simulink model "DZ_DSMC4"  (R2021b)
settings: Solver=FixedStepAuto  StartTime=0.0  StopTime=30  FixedStep=Ts  MaxStep=0.015  RelTol=1e-3  EnableMultiTasking=on
PreLoadFcn:
  | if ~exist('sim_HIL')
  |     sim_HIL=false;
  | end
  | if ~exist('usefilter')
  |     usefilter=false;
  | end
InitFcn:
  | load motorModel.mat
  | load expsetup
undefined symbols (not defined in the file): Cs, dels, etas, gamms, mModel, N, qTs, Ts, vphis, xiTs
settings Model: DataDictionary=MotorInfo.sldd  CodeVerificationMode=processor-in-the-loop (pil)  ExtModeTrigDuration=2  Creator=khoi  LastModifiedBy=khoi
settings SolverCC: AlgebraicLoopSolver=TrustRegion
settings DataIOCC: ExternalInput=i1, i2  SaveOutput=off  SaveTime=off
settings OptimizationCC: UseDivisionForNetSlopeComputation=on  GainParamInheritBuiltInType=on  UseFloatMulNetSlope=on  DefaultUnderspecifiedDataType=single  StrengthReduction=on  BitwiseOrLogicalOp=Bitwise operator  PassReuseOutputArgsAs=Individual arguments  ZeroExternalMemoryAtStartup=off  ZeroInternalMemoryAtStartup=off  EfficientFloat2IntCast=on  LifeSpan=1  MaxStackSize=64  OptimizeBlockOrder=speed  OptimizationPriority=Speed  OptimizationCustomize=off  MultiThreadedLoops=on  EfficientTunableParamExpr=on
settings DebuggingCC: SignalInfNanChecking=error  AlgebraicLoopMsg=none  ParameterTunabilityLossMsg=error  UniqueDataStoreMsg=error  AssertControl=DisableAll  StrictBusMsg=ErrorOnBusTreatedAsVector  SFUndirectedBroadcastEventsDiag=error  SFMachineParentedDataDiag=warning
settings HardwareCC: ProdBitPerInt=16  ProdBitPerPointer=16  ProdBitPerSizeT=16  ProdBitPerPtrDiffT=16  ProdLargestAtomicFloat=None  ProdWordSize=8  ProdHWDeviceType=Atmel->AVR
settings ModelReferenceCC: PropagateVarSize=During execution
settings SFSimCC: CompileTimeRecursionLimit=0  EnableRuntimeRecursion=off  MATLABDynamicMemAlloc=off
settings RTWCC: Description=Embedded Coder  SystemTargetFile=ert.tlc  HardwareBoard=Arduino Mega 2560  TemplateMakefile=ert_default_tmf  Toolchain=Arduino AVR  BuildConfiguration=Faster Runs
settings CodeAppCC: ForceParamTrailComments=on  IgnoreCustomStorageClasses=off  IgnoreTestpoints=on  OperatorAnnotations=on  SimulinkDataObjDesc=on  SFDataObjDesc=on  MATLABFcnDesc=on  InsertBlockDesc=on
settings ERTTargetCC: TargetLangStandard=C99 (ISO)  CodeReplacementLibrary=GNU C99 extensions  UtilityFuncGeneration=Shared location  SupportNonFinite=off  SupportComplex=off  ParenthesesLevel=Maximum  CastingMode=Standards  GenerateSharedConstants=off  ExtModeTransport=3  ExtModeStaticAlloc=on  ExtModeStaticAllocSize=2048  ExtModeMexFile=ext_xcp  ExtModeIntrfLevel=Level2 - Open  EnableSignedLeftShifts=off  EnableSignedRightShifts=off
settings ConfigComp: CovScope=ReferencedModels

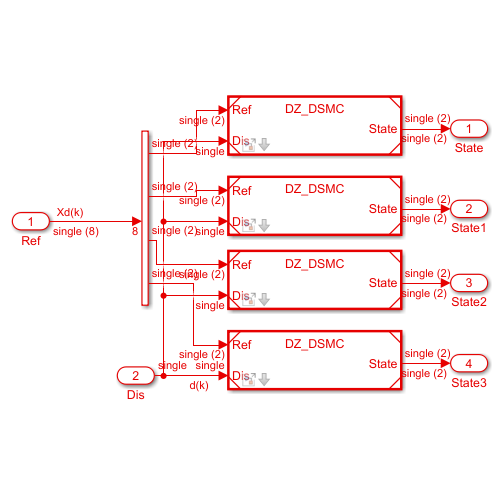
[thumbnail: Simulink's stored preview of the top-level diagram]
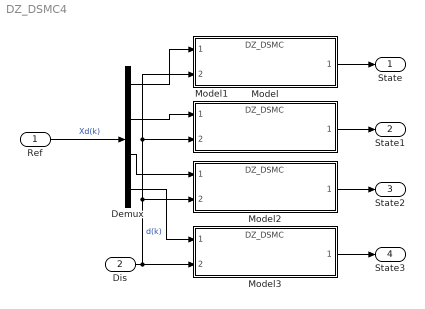
== system DZ_DSMC4 ==
  Ref : Inport  OutDataTypeStr=single  PortDimensions=8
  Dis : Inport  Port=2  OutDataTypeStr=single  PortDimensions=1
  Demux : Demux
  Model : ModelReference  ModelNameDialog=DZ_DSMC.slx  SimulationMode=Normal  ModelReferenceVersion=4.50  mask{Phi=mModel{1,3}.A, Gam=mModel{1,3}.B, C=Cs(1,:), qT=qTs(1), xiT=xiTs(1), del=dels(1), vphi=vphis(1), gamm=gamms(1), eta=etas(1), Ts=Ts, N=N}
      mask prompts: Phi "state A"; Gam "state B"; C "Sliding vector"; del "delta"; gamm "gamma"
  Model1 : ModelReference  ModelNameDialog=DZ_DSMC.slx  SimulationMode=Normal  ModelReferenceVersion=4.50  mask{Phi=mModel{2,3}.A, Gam=mModel{2,3}.B, C=Cs(2,:), qT=qTs(2), xiT=xiTs(2), del=dels(2), vphi=vphis(2), gamm=gamms(2), eta=etas(2), Ts=Ts, N=N}
      mask prompts: Phi "state A"; Gam "state B"; C "Sliding vector"; del "delta"; gamm "gamma"
  Model2 : ModelReference  ModelNameDialog=DZ_DSMC.slx  SimulationMode=Normal  ModelReferenceVersion=4.50  mask{Phi=mModel{3,3}.A, Gam=mModel{3,3}.B, C=Cs(3,:), qT=qTs(3), xiT=xiTs(3), del=dels(3), vphi=vphis(3), gamm=gamms(3), eta=etas(3), Ts=Ts, N=N}
      mask prompts: Phi "state A"; Gam "state B"; C "Sliding vector"; del "delta"; gamm "gamma"
  Model3 : ModelReference  ModelNameDialog=DZ_DSMC.slx  SimulationMode=Normal  ModelReferenceVersion=4.50  mask{Phi=mModel{4,3}.A, Gam=mModel{4,3}.B, C=Cs(4,:), qT=qTs(4), xiT=xiTs(4), del=dels(4), vphi=vphis(4), gamm=gamms(4), eta=etas(4), Ts=Ts, N=N}
      mask prompts: Phi "state A"; Gam "state B"; C "Sliding vector"; del "delta"; gamm "gamma"
  State : Outport  OutDataTypeStr=single  PortDimensions=2
  State1 : Outport  Port=2  OutDataTypeStr=single  PortDimensions=2
  State2 : Outport  Port=3  OutDataTypeStr=single  PortDimensions=2
  State3 : Outport  Port=4  OutDataTypeStr=single  PortDimensions=2
  wires:
  Ref/1 -> Demux/1  "Xd(k)"
  Model3/1 -> State3/1
  Demux/2 -> Model1/1
  Model2/1 -> State2/1
  Demux/1 -> Model/1
  Demux/3 -> Model2/1
  Model/1 -> State/1
  Model1/1 -> State1/1
  Demux/4 -> Model3/1
  Dis/1 -> Model1/2, Model/2, Model2/2, Model3/2  "d(k)"
